simulink model "uav2_model"  (R2015b)
settings: Solver=FixedStepAuto  SolverMode=SingleTasking  StartTime=t_s  StopTime=t_e  FixedStep=dt  RelTol=1e-3
values from neighbouring files (symbols this model uses):
  A = [ ... (first row only)    [uav2_data.m]
  B = [ ... (first row only)    [uav2_data.m]
  C = eye(4,4)    [uav2_data.m]
  D = zeros(4,1)    [uav2_data.m]
  dt = 0.1    [main.m]
  init = [0.01 0 0 0]    [main.m]
settings Model: Creator=yakov  LastModifiedBy=Administrator
settings DataIOCC: LimitDataPoints=off  ReturnWorkspaceOutputs=on
settings OptimizationCC: DefaultParameterBehavior=Inlined  OptimizeModelRefInitCode=on
settings DebuggingCC: AllowSymbolicDim=on  SFUnexpectedBacktrackingDiag=error  SFNoUnconditionalDefaultTransitionDiag=error
settings HardwareCC: TargetIntDivRoundTo=Zero  TargetEndianess=LittleEndian  TargetHWDeviceType=MATLAB Host  ProdEqTarget=off
settings ModelReferenceCC: PropagateSignalLabelsOutOfModel=on
settings SFSimCC: SimUseLocalCustomCode=on
settings RTWCC: SystemTargetFile=ert_shrlib.tlc  GenCodeOnly=on  TemplateMakefile=ert_default_tmf  Description=Embedded Coder (host-based shared library target)  RTWUseLocalCustomCode=on
settings CodeAppCC: IgnoreCustomStorageClasses=off
settings STFCustomTargetCC: GenerateSampleERTMain=on  ParMdlRefBuildCompliant=on  CompOptLevelCompliant=on  ConcurrentExecutionCompliant=off  GeneratePreprocessorConditionals=Use local settings  CombineOutputUpdateFcns=on  ERTCustomFileBanners=on  SupportNonInlinedSFcns=off  MATLABClassNameForMDSCustomization=Simulink.SoftwareTarget.ERTCustomization  ModelStepFunctionPrototypeControlCompliant=on  CPPClassGenCompliant=off  GRTInterface=off  UseToolchainInfoCompliant=on  SystemTargetFile=ert_shrlib.tlc
settings ERTTargetCC: GenerateSampleERTMain=on  ConcurrentExecutionCompliant=off  ERTFirstTimeCompliant=off  SupportContinuousTime=on  CPPClassGenCompliant=off  InlinedParameterPlacement=NonHierarchical  ERTCustomFileTemplate=example_file_process.tlc
settings ConfigComp: CovMetricSettings=dwe  CovSaveCumulativeToWorkspaceVar=off  CovSaveSingleToWorkspaceVar=off  CovModelRefEnable=Off  CovExternalEMLEnable=on

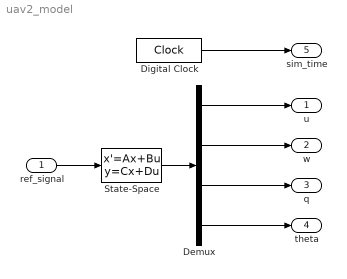
== system uav2_model ==
  ref_signal : Inport
  Demux : Demux
  Digital Clock : DigitalClock  SampleTime=dt
  State-Space : StateSpace  A=A  B=B  C=C  D=D  X0=init  ContinuousStateAttributes={'u','w', 'q', 'theta'}
  u : Outport
  w : Outport  Port=2
  q : Outport  Port=3
  theta : Outport  Port=4
  "sim_time " : Outport  Port=5
  wires:
  ref_signal/1 -> State-Space/1
  Demux/2 -> w/1
  State-Space/1 -> Demux/1
  Demux/1 -> u/1
  Demux/3 -> q/1
  Demux/4 -> theta/1
  Digital Clock/1 -> "sim_time "/1
